simulink model "Kalman_Filter_Simulink_Example"  (R2018a)
settings: Solver=FixedStepAuto  StartTime=0.0  StopTime=30  FixedStep=.01  RelTol=1e-3
values from neighbouring files (symbols this model uses):
  g = 9.81    [Kalman_Filter_Simulink_Example_params.m]
  l = 0.5    [Kalman_Filter_Simulink_Example_params.m]
  P0 = [1e-6 0; 0 1e-6]    [Kalman_Filter_Simulink_Example_params.m]
  Q = 1e-4    (= 0.0001)    [Kalman_Filter_Simulink_Example_params.m]
  R = 1e-3    (= 0.001)    [Kalman_Filter_Simulink_Example_params.m]
  theta0 = pi/4    (= 0.785398163397)    [Kalman_Filter_Simulink_Example_params.m]
  Ts = 0.01    [Kalman_Filter_Simulink_Example_params.m]
undefined symbols (not defined in the file or in its folder): Q0, R0
libraries: simulink x7, dspmtrx3 x5, sharedTrackingLibrary x1, Meldas_Library x1
settings Model: Creator=mulusoy  LastModifiedBy=hussein
settings OptimizationCC: DefaultParameterBehavior=Inlined  PassReuseOutputArgsAs=Individual arguments
settings DebuggingCC: ParameterTunabilityLossMsg=error
settings SFSimCC: MATLABDynamicMemAlloc=off
settings RTWCC: SystemTargetFile=ert.tlc  TemplateMakefile=ert_default_tmf  GenerateReport=on  IncludeHyperlinkInReport=on  LaunchReport=on  GenerateTraceInfo=on  GenerateTraceReport=on  GenerateTraceReportSl=on  GenerateTraceReportSf=on  GenerateTraceReportEml=on  CheckMdlBeforeBuild=Warning
settings CodeAppCC: GenerateComments=off  IgnoreCustomStorageClasses=off  SimulinkBlockComments=off
settings ERTTargetCC: TargetLangStandard=C99 (ISO)  GenerateSampleERTMain=on  InlinedParameterPlacement=NonHierarchical  ERTCustomFileTemplate=example_file_process.tlc
settings SimscapeCC: SimscapeNormalizeSystem=off

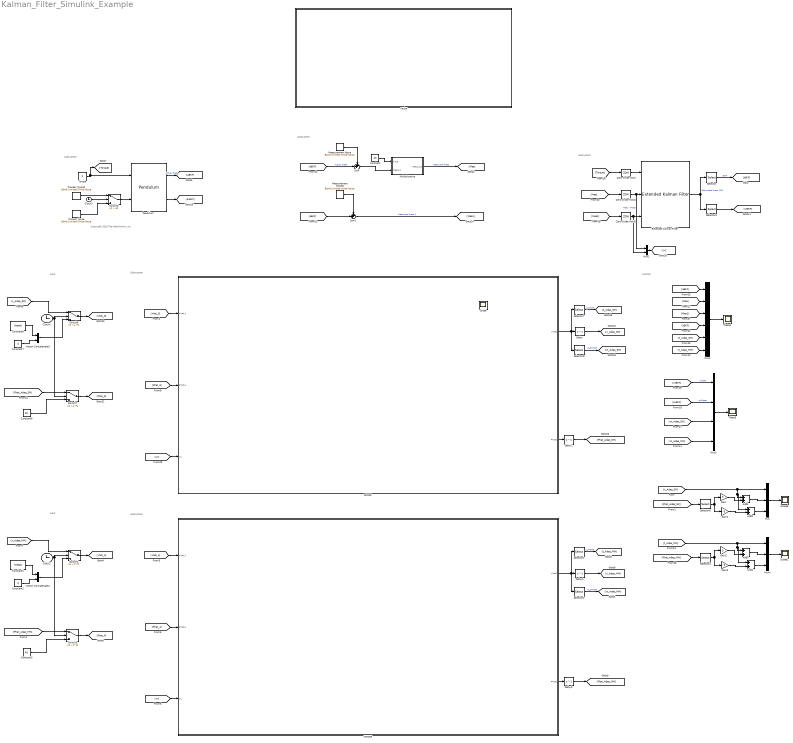
== system Kalman_Filter_Simulink_Example ==
  note: Subsystem
  note: Subsystem
  note: Subsystem
  note: Monitor
  note: Input
  note: Subsystem
  note: Input
  note: Subsystem
  note: Copyright 2018 The MathWorks, Inc.
  Add{1..4} (4 alike) : Sum
  Clock2 : Clock
      settings: Decimation=1000
  Clock3 : Clock
  Clock4 : Clock
      settings: Decimation=1000
  Constant : Constant  Value=20
  Constant1 : Constant  Value=theta0
  Constant2 : Constant  Value=0
  Constant3 : Constant  Value=P0
  Constant6 : Constant  Value=theta0
  Constant7 : Constant  Value=0
  Constant8 : Constant  Value=P0
  Delay{,1..3} (4 alike) : Delay  DelayLength=1
  Extended Kalman Filter : sharedTrackingLibrary/Extended Kalman Filter  StateTransitionFcn=myStateTransitionFcn  HasStateTransitionJacobianFcn=off  HasAdditiveProcessNoise=Additive  ProcessNoise=diag([0,Q0])  HasTimeVaryingProcessNoise=off  HasStateTransitionFcnExtraArgument=1  InitialState=[pi/4 0]  InitialStateCovariance=1e-6  MeasurementFcn1=myMeasurementFcn  HasMeasurementJacobianFcn1=off  HasMeasurementEnablePort1=off  HasAdditiveMeasurementNoise1=Additive  MeasurementNoise1=R0  HasTimeVaryingMeasurementNoise1=off  HasMeasurementFcnExtraArgument1=0  MeasurementFcn2=myMeasurementFcn  HasMeasurementJacobianFcn2=off  HasMeasurementEnablePort2=off  HasAdditiveMeasurementNoise2=Additive  MeasurementNoise2=R0  HasTimeVaryingMeasurementNoise2=off  HasMeasurementFcnExtraArgument2=0  MeasurementFcn3=myMeasurementFcn  HasMeasurementJacobianFcn3=off  HasMeasurementEnablePort3=off  HasAdditiveMeasurementNoise3=Additive  MeasurementNoise3=1  HasTimeVaryingMeasurementNoise3=off  HasMeasurementFcnExtraArgument3=0  MeasurementFcn4=myMeasurementFcn  HasMeasurementJacobianFcn4=off  HasMeasurementEnablePort4=off  HasAdditiveMeasurementNoise4=Additive  MeasurementNoise4=1  HasTimeVaryingMeasurementNoise4=off  HasMeasurementFcnExtraArgument4=0  MeasurementFcn5=myMeasurementFcn  HasMeasurementJacobianFcn5=off  HasMeasurementEnablePort5=off  HasAdditiveMeasurementNoise5=Additive  MeasurementNoise5=1  HasTimeVaryingMeasurementNoise5=off  HasMeasurementFcnExtraArgument5=0  EnableMultirate=off  StateTransitionFcnSampleTime=1  MeasurementFcn1SampleTime=1  MeasurementFcn2SampleTime=1  MeasurementFcn3SampleTime=1  MeasurementFcn4SampleTime=1  MeasurementFcn5SampleTime=1  UseCurrentEstimator=on  OutputStateCovariance=off  DataType=double  SampleTime=Ts  NumberOfMeasurements=2
      settings: SourceProductName=Control System Toolbox  SourceProductBaseCode=CT
  Faults : Subsystem
  Gain : Gain  Gain=3
  Gain1 : Gain  Gain=-3
  Gain2 : Gain  Gain=3
  Gain3 : Gain  Gain=-3
  MMNSF : Subsystem
  Measurement Noise : simulink/Sources/Band-Limited White Noise  Cov=R*Ts  Ts=Ts  seed=[12347]
  Measurement Noise3 : simulink/Sources/Band-Limited White Noise  Cov=R*Ts  Ts=Ts  seed=[12347]
  Multiplicative : Subsystem
  Mux : Mux  Inputs=3
  Mux1 : Mux  Inputs=2
  Mux2 : Mux  Inputs=6
  Mux3 : Mux
  Mux4 : Mux  Inputs=3
  Pendulum : Meldas_Library/Pendulum  theta_0=pi/3  theta_dot_0=0
      link override Revolute Joint: SenseVelocity=on
  Process Noise2 : simulink/Sources/Band-Limited White Noise  Cov=Q*Ts*1000  Ts=Ts  seed=[12347]
  Process Noise : simulink/Sources/Band-Limited White Noise  Cov=0  Ts=Ts  seed=[23341]
  SMNSF : Subsystem
  Scope1 : Scope
  Scope5 : Scope
  Selector : Selector  InputPortWidth=2  IndexOptions=Index vector (dialog)  Indices=1  OutputSizes=1
  Selector1 : Selector  InputPortWidth=2  IndexOptions=Index vector (dialog)  Indices=1  OutputSizes=1
  Selector2 : Selector  InputPortWidth=2  IndexOptions=Index vector (dialog)  Indices=2  OutputSizes=1
  Selector3 : Selector  InputPortWidth=2  IndexOptions=Index vector (dialog)  Indices=2  OutputSizes=1
  Selector4 : Selector  NumberOfDimensions=2  InputPortWidth=3  IndexOptions=Index vector (dialog),Index vector (dialog)  Indices=1,1  OutputSizes=1,1
  Selector6 : Selector  NumberOfDimensions=2  InputPortWidth=3  IndexOptions=Index vector (dialog),Index vector (dialog)  Indices=1,1  OutputSizes=1,1
  Selector7 : Selector  InputPortWidth=2  IndexOptions=Index vector (dialog)  Indices=1  OutputSizes=1
  Selector8 : Selector  InputPortWidth=2  IndexOptions=Index vector (dialog)  Indices=2  OutputSizes=1
  Sum : Sum  Inputs=++|
  Sum1 : Sum  Inputs=++|
  Switch{1,3,6..7} (4 alike) : Switch  Threshold=Ts
  Switch5 : Switch  Criteria=u2 > Threshold  Threshold=40
  Theta4 : Scope
  Theta5 : Scope
  Torque : Constant  Value=0
  Vector Concatenate1 : Concatenate
  Vector Concatenate2 : Concatenate
  Zero-Order Hold : ZeroOrderHold  SampleTime=Ts
  Zero-Order Hold1 : ZeroOrderHold  SampleTime=Ts
  Zero-Order Hold2 : ZeroOrderHold  SampleTime=Ts
  Scope : Scope
  wires:
  [Mea] -> Mux2/2
  [vtEKF] -> Mux3/1  "vtheta"
  Mux3/1 -> Theta5/1
  Mux2/1 -> Theta4/1
  [avEKF] -> Mux3/2  "aVtheta"
  [tEKF] -> Mux2/4
  [aEKF] -> Mux2/1
  [Phat_Adap_SM] -> Selector6/1
  [t_Adap_SM] -> Add2/1, Add1/1, Mux/1
  Selector6/1 -> Gain/1, Gain1/1
  Gain/1 -> Add1/2
  Add1/1 -> Mux/2
  Gain1/1 -> Add2/2
  Add2/1 -> Mux/3
  Mux/1 -> Scope5/1
  Selector7/1 -> [t_Adap_SM]  "t_SMNSF"
  Vector Concatenate2/1 -> Switch6/3
  SMNSF/2(Phat1) -> Delay1/1
  Clock4/1 -> Switch7/2, Switch6/2
  Constant7/1 -> Vector Concatenate2/2
  [x_Adap_SM] -> Switch6/1
  SMNSF/1(xhat1) -> Selector8/1, Selector7/1, Delay/1
  [Phat_3] -> SMNSF/2(Phat_1)
  Constant6/1 -> Vector Concatenate2/1
  [Phat_Adap_SM] -> Switch7/1
  Switch6/1 -> [xhat_3]
  Constant8/1 -> Switch7/3
  Selector8/1 -> [vt_Adap_SM]  "vt_SMNSF"
  Switch7/1 -> [Phat_3]
  [yv] -> SMNSF/3(y1)
  [xhat_3] -> SMNSF/1(xhat_1)
  [t_Adap_SM] -> Mux2/5
  Delay/1 -> [x_Adap_SM]
  Delay1/1 -> [Phat_Adap_SM]
  [Mea1] -> Mux2/3
  [vt_Adap_SM] -> Mux3/3
  Selector1/1 -> [t_Adap_MM]  "t_SMNSF"
  Delay2/1 -> [x_Adap_MM]
  MMNSF/2(Phat1) -> Delay3/1
  Vector Concatenate1/1 -> Switch1/3
  [xhat_4] -> MMNSF/1(xhat_1)
  Selector2/1 -> [vt_Adap_MM]  "vt_SMNSF"
  Switch1/1 -> [xhat_4]
  Constant3/1 -> Switch3/3
  Switch3/1 -> [Phat_4]
  [Phat_4] -> MMNSF/2(Phat_1)
  Constant1/1 -> Vector Concatenate1/1
  [Phat_Adap_MM] -> Switch3/1
  MMNSF/1(xhat1) -> Selector2/1, Selector1/1, Delay2/1
  [x_Adap_MM] -> Switch1/1
  Clock2/1 -> Switch3/2, Switch1/2
  Constant2/1 -> Vector Concatenate1/2
  [yv] -> MMNSF/3(y1)
  Delay3/1 -> [Phat_Adap_MM]
  [t_Adap_MM] -> Mux2/6
  [vt_Adap_MM] -> Mux3/4
  [aEKF] -> Sum/2  "Actual theta"
  [aEKF] -> Sum1/2
  Measurement Noise/1 -> Sum/1
  Measurement Noise3/1 -> Sum1/1
  Sum1/1 -> [Mea1]  "Measured theta 2"
  Multiplicative/1(Meas_out) -> [Mea]  "Measured theta"
  Clock3/1 -> Switch5/2
  Process Noise/1 -> Switch5/3
  Pendulum/2 -> [avEKF]
  Pendulum/1 -> [aEKF]  "Actual theta"
  Torque/1 -> Pendulum/1, [Torque]
  Switch5/1 -> Pendulum/2
  [Mea1] -> Zero-Order Hold2/1
  [Torque] -> Zero-Order Hold/1
  Selector/1 -> [tEKF]  "tEKF"
  Zero-Order Hold/1 -> Extended Kalman Filter/1
  Mux1/1 -> [yv]
  Selector3/1 -> [vtEKF]
  Zero-Order Hold2/1 -> Mux1/2, Extended Kalman Filter/3
  Extended Kalman Filter/1 -> Selector/1, Selector3/1  "Estimated theta  EKF"
  [Mea] -> Zero-Order Hold1/1
  Zero-Order Hold1/1 -> Mux1/1, Extended Kalman Filter/2  "Meas  Theta"
  Process Noise2/1 -> Switch5/1
  Selector4/1 -> Gain2/1, Gain3/1
  Add3/1 -> Mux4/2
  Gain3/1 -> Add4/2
  [Phat_Adap_MM] -> Selector4/1
  [t_Adap_MM] -> Add4/1, Add3/1, Mux4/1
  Gain2/1 -> Add3/2
  Add4/1 -> Mux4/3
  Mux4/1 -> Scope1/1
  Constant/1 -> Multiplicative/1(Time)
  Sum/1 -> Multiplicative/2("Meas_in ")

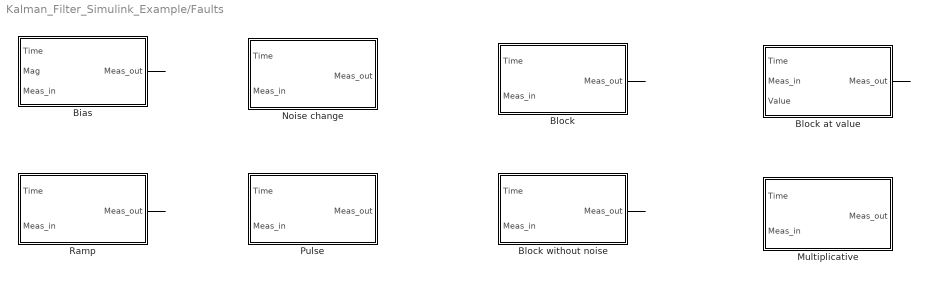
== system Kalman_Filter_Simulink_Example/Faults ==
  Bias : Subsystem
  Block : Subsystem
  Block at value : Subsystem
  Block without noise : Subsystem
  Multiplicative : Subsystem
  Noise change : Subsystem
  Pulse : Subsystem
  Ramp : Subsystem
  wires:
  ? -> Block/2("Meas_in ")
  ? -> Block at value/2("Meas_in ")
  Bias/1(Meas_out) -> ?
  ? -> Ramp/2("Meas_in ")
  ? -> Block without noise/2("Meas_in ")
  Block at value/1(Meas_out) -> ?
  ? -> Bias/1(Time)
  ? -> Block at value/1(Time)
  ? -> Bias/2(Mag)
  Block/1(Meas_out) -> ?
  ? -> Block at value/3(Value)
  Block without noise/1(Meas_out) -> ?
  ? -> Block/1(Time)
  ? -> Block without noise/1(Time)
  Ramp/1(Meas_out) -> ?
  ? -> Ramp/1(Time)
  ? -> Bias/3("Meas_in ")

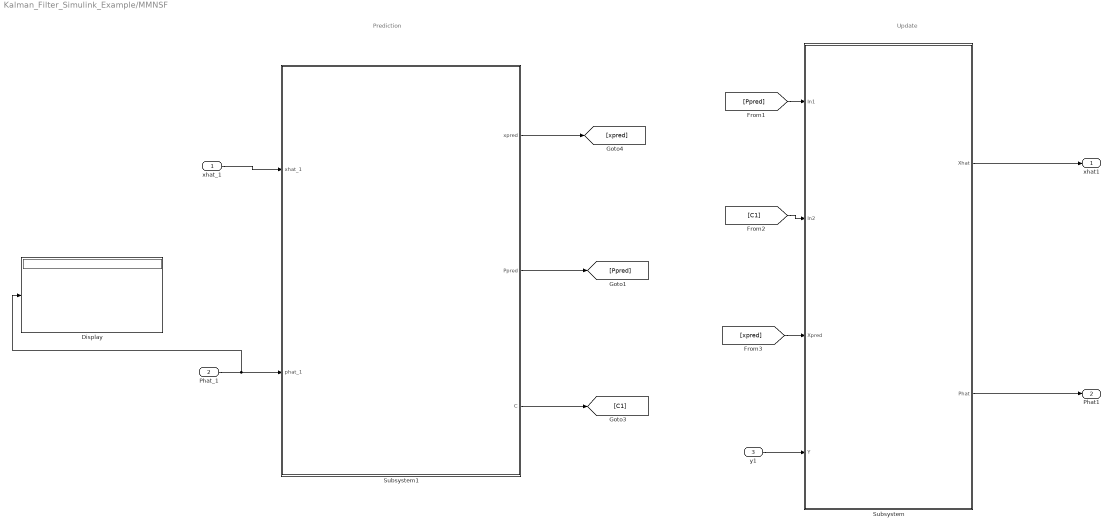
== system Kalman_Filter_Simulink_Example/MMNSF ==
  note: Update
  note: Prediction
  xhat_1 : Inport
  Phat_1 : Inport  Port=2
  y1 : Inport  Port=3
  Display : Display
  Subsystem : Subsystem
  Subsystem1 : Subsystem
  xhat1 : Outport
  Phat1 : Outport  Port=2
  wires:
  [Ppred] -> Subsystem/1(In1)
  Subsystem/1(Xhat) -> xhat1/1
  y1/1 -> Subsystem/4("Y ")
  Subsystem1/1(xpred) -> [xpred]
  Subsystem/2("Phat ") -> Phat1/1
  [C1] -> Subsystem/2(In2)
  Phat_1/1 -> Subsystem1/2(phat_1), Display/1
  [xpred] -> Subsystem/3(Xpred)
  xhat_1/1 -> Subsystem1/1(xhat_1)
  Subsystem1/2(Ppred) -> [Ppred]
  Subsystem1/3("C ") -> [C1]

== system Kalman_Filter_Simulink_Example/Multiplicative ==
  Time : Inport
  "Meas_in " : Inport  Port=2
  Clock : Clock
  Gain : Gain  Gain=2
  Sum : Sum  Inputs=+-
  Switch : Switch  Criteria=u2 > Threshold
  Meas_out : Outport
  wires:
  Switch/1 -> Meas_out/1
  Sum/1 -> Switch/2
  Clock/1 -> Sum/1
  Time/1 -> Sum/2
  "Meas_in "/1 -> Gain/1, Switch/3
  Gain/1 -> Switch/1

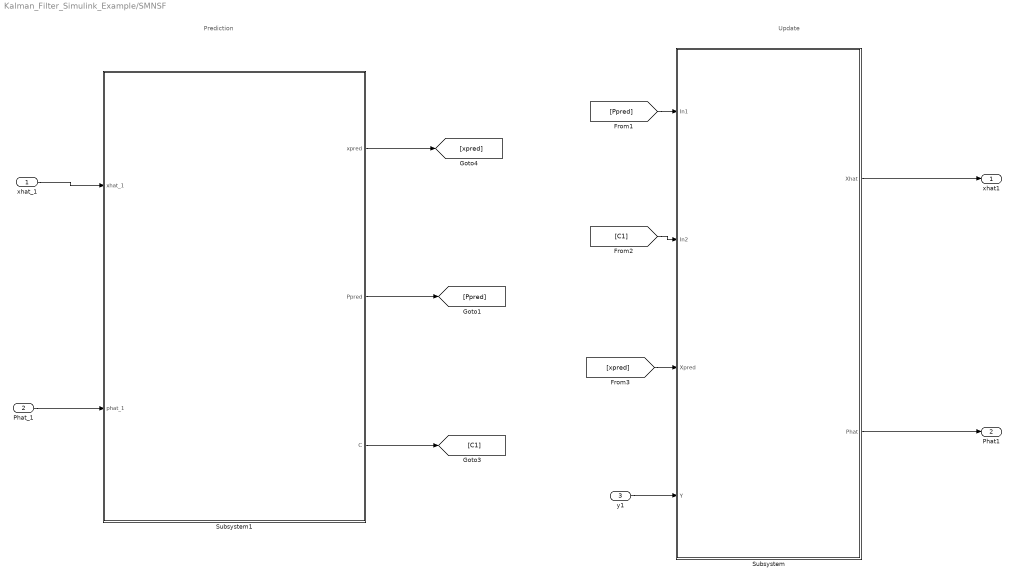
== system Kalman_Filter_Simulink_Example/SMNSF ==
  note: Update
  note: Prediction
  xhat_1 : Inport
  Phat_1 : Inport  Port=2
  y1 : Inport  Port=3
  Subsystem : Subsystem
  Subsystem1 : Subsystem
  xhat1 : Outport
  Phat1 : Outport  Port=2
  wires:
  [Ppred] -> Subsystem/1(In1)
  Subsystem/1(Xhat) -> xhat1/1
  y1/1 -> Subsystem/4("Y ")
  Subsystem1/1(xpred) -> [xpred]
  Subsystem/2("Phat ") -> Phat1/1
  [C1] -> Subsystem/2(In2)
  Phat_1/1 -> Subsystem1/2(phat_1)
  [xpred] -> Subsystem/3(Xpred)
  xhat_1/1 -> Subsystem1/1(xhat_1)
  Subsystem1/2(Ppred) -> [Ppred]
  Subsystem1/3("C ") -> [C1]

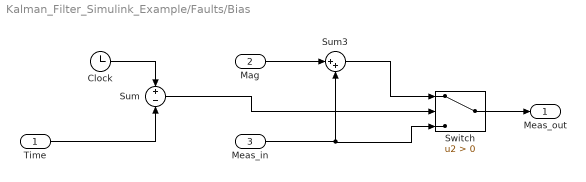
== system Kalman_Filter_Simulink_Example/Faults/Bias ==
  Time : Inport
  Mag : Inport  Port=2
  "Meas_in " : Inport  Port=3
  Clock : Clock
  Sum : Sum  Inputs=+-
  Sum3 : Sum  Inputs=|++
  Switch : Switch  Criteria=u2 > Threshold
  Meas_out : Outport
  wires:
  Sum/1 -> Switch/2
  Clock/1 -> Sum/1
  Switch/1 -> Meas_out/1
  Time/1 -> Sum/2
  Sum3/1 -> Switch/1
  Mag/1 -> Sum3/1
  "Meas_in "/1 -> Sum3/2, Switch/3

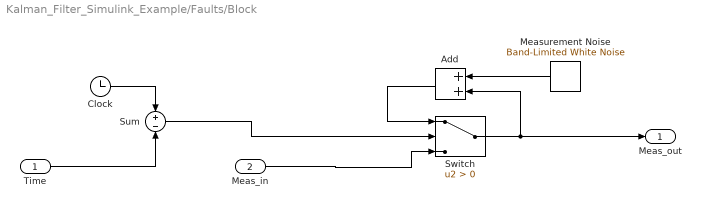
== system Kalman_Filter_Simulink_Example/Faults/Block ==
  Time : Inport
  "Meas_in " : Inport  Port=2
  Add : Sum
  Clock : Clock
  Measurement Noise : simulink/Sources/Band-Limited White Noise  Cov=R*Ts  Ts=Ts  seed=[12347]
  Sum : Sum  Inputs=+-
  Switch : Switch  Criteria=u2 > Threshold
  Meas_out : Outport
  wires:
  "Meas_in "/1 -> Switch/3
  Time/1 -> Sum/2
  Switch/1 -> Add/2, Meas_out/1
  Clock/1 -> Sum/1
  Sum/1 -> Switch/2
  Add/1 -> Switch/1
  Measurement Noise/1 -> Add/1

== system Kalman_Filter_Simulink_Example/Faults/Block at value ==
  Time : Inport
  "Meas_in " : Inport  Port=2
  Value : Inport  Port=3
  Clock : Clock
  Sum : Sum  Inputs=+-
  Switch : Switch  Criteria=u2 > Threshold
  Meas_out : Outport
  wires:
  "Meas_in "/1 -> Switch/3
  Time/1 -> Sum/2
  Clock/1 -> Sum/1
  Sum/1 -> Switch/2
  Switch/1 -> Meas_out/1
  Value/1 -> Switch/1

== system Kalman_Filter_Simulink_Example/Faults/Block without noise ==
  Time : Inport
  "Meas_in " : Inport  Port=2
  Clock : Clock
  Sum : Sum  Inputs=+-
  Switch : Switch  Criteria=u2 > Threshold
  Meas_out : Outport
  wires:
  Switch/1 -> Switch/1, Meas_out/1
  Sum/1 -> Switch/2
  Clock/1 -> Sum/1
  Time/1 -> Sum/2
  "Meas_in "/1 -> Switch/3

== system Kalman_Filter_Simulink_Example/Faults/Multiplicative ==
  Time : Inport
  "Meas_in " : Inport  Port=2
  Clock : Clock
  Gain : Gain  Gain=1.1
  Sum : Sum  Inputs=+-
  Switch : Switch  Criteria=u2 > Threshold
  Meas_out : Outport
  wires:
  Switch/1 -> Meas_out/1
  Sum/1 -> Switch/2
  Clock/1 -> Sum/1
  Time/1 -> Sum/2
  "Meas_in "/1 -> Gain/1, Switch/3
  Gain/1 -> Switch/1

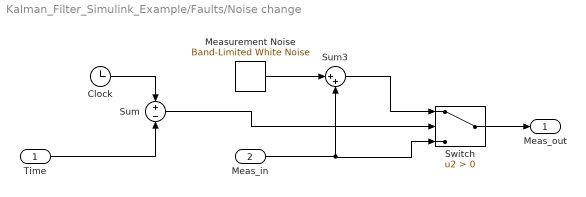
== system Kalman_Filter_Simulink_Example/Faults/Noise change ==
  Time : Inport
  "Meas_in " : Inport  Port=2
  Clock : Clock
  Measurement Noise : simulink/Sources/Band-Limited White Noise  Cov=0.01  Ts=Ts  seed=[12347]
  Sum : Sum  Inputs=+-
  Sum3 : Sum  Inputs=|++
  Switch : Switch  Criteria=u2 > Threshold
  Meas_out : Outport
  wires:
  "Meas_in "/1 -> Switch/3, Sum3/2
  Measurement Noise/1 -> Sum3/1
  Sum3/1 -> Switch/1
  Time/1 -> Sum/2
  Switch/1 -> Meas_out/1
  Clock/1 -> Sum/1
  Sum/1 -> Switch/2

== system Kalman_Filter_Simulink_Example/Faults/Pulse ==
  Time : Inport
  "Meas_in " : Inport  Port=2
  Clock : Clock
  Pulse Generator : DiscretePulseGenerator  Amplitude=0.1  Period=10  PulseWidth=5  SampleTime=0.01
  Sum : Sum  Inputs=+-
  Sum3 : Sum  Inputs=|++
  Switch : Switch  Criteria=u2 > Threshold
  Meas_out : Outport
  wires:
  Sum/1 -> Switch/2
  Clock/1 -> Sum/1
  Switch/1 -> Meas_out/1
  Time/1 -> Sum/2
  Sum3/1 -> Switch/1
  Pulse Generator/1 -> Sum3/1
  "Meas_in "/1 -> Sum3/2, Switch/3

== system Kalman_Filter_Simulink_Example/Faults/Ramp ==
  Time : Inport
  "Meas_in " : Inport  Port=2
  Clock : Clock
  Ramp : simulink/Sources/Ramp  slope=0.1  start=10  InitialOutput=0
  Sum : Sum  Inputs=+-
  Sum3 : Sum  Inputs=|++
  Switch : Switch  Criteria=u2 > Threshold
  Meas_out : Outport
  wires:
  "Meas_in "/1 -> Switch/3, Sum3/2
  Ramp/1 -> Sum3/1
  Sum3/1 -> Switch/1
  Time/1 -> Sum/2
  Switch/1 -> Meas_out/1
  Clock/1 -> Sum/1
  Sum/1 -> Switch/2

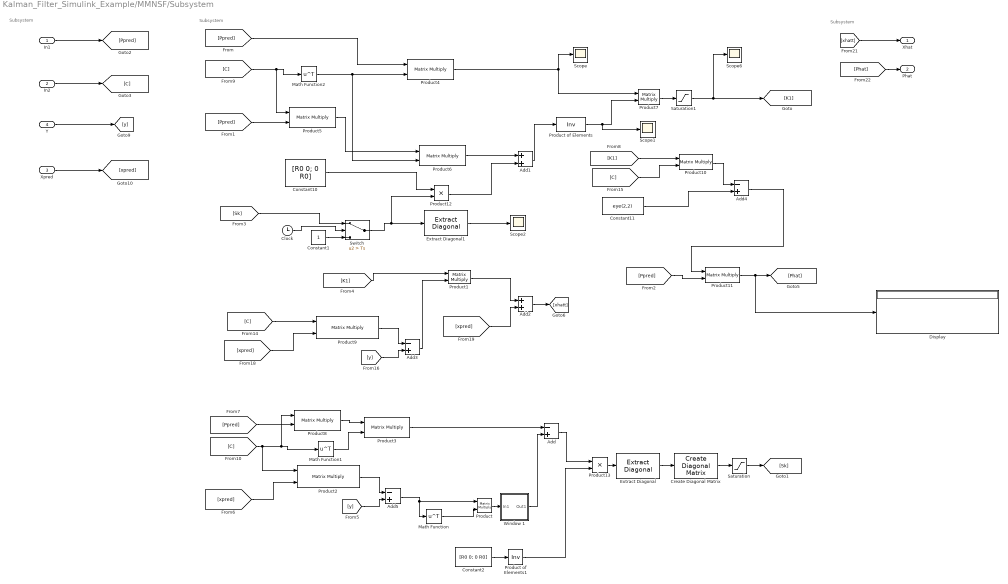
== system Kalman_Filter_Simulink_Example/MMNSF/Subsystem ==
  note: Subsystem
  note: Subsystem
  note: Subsystem
  In1 : Inport
  In2 : Inport  Port=2
  Xpred : Inport  Port=3
  "Y " : Inport  Port=4
  Add{,3..5} (4 alike) : Sum  Inputs=-+
  Add1 : Sum
  Add2 : Sum
  Clock : Clock
  Constant1 : Constant
  Constant10 : Constant  Value=[R0 0; 0 R0]
  Constant11 : Constant  Value=eye(2,2)
  Constant2 : Constant  Value=[R0 0; 0 R0]
  Create Diagonal Matrix : dspmtrx3/Create Diagonal Matrix
      settings: SourceProductName=DSP System Toolbox  SourceProductBaseCode=DS
  Display : Display
  Extract Diagonal : dspmtrx3/Extract Diagonal
      settings: SourceProductName=DSP System Toolbox  SourceProductBaseCode=DS
  Extract Diagonal1 : dspmtrx3/Extract Diagonal
      settings: SourceProductName=DSP System Toolbox  SourceProductBaseCode=DS
  Math Function : Math  Operator=transpose  SaturateOnIntegerOverflow=on
  Math Function1 : Math  Operator=transpose  SaturateOnIntegerOverflow=on
  Math Function2 : Math  Operator=transpose  SaturateOnIntegerOverflow=on
  Product{,1..11} (12 alike) : Product  Multiplication=Matrix(*)
  Product of Elements : Product  Inputs=/  Multiplication=Matrix(*)
  Product of Elements1 : Product  Inputs=/  Multiplication=Matrix(*)
  Product12 : Product
  Product13 : Product
  Saturation : Saturate  UpperLimit=1000  LowerLimit=1
  Saturation1 : Saturate  UpperLimit=1  LowerLimit=0
  Scope{,1..2,6} (4 alike) : Scope
  Switch : Switch  Criteria=u2 > Threshold  Threshold=Ts
  Window 1 : Subsystem
  Xhat : Outport  PortDimensions=[2,1]
  "Phat " : Outport  Port=2
  wires:
  Add2/1 -> [xhatt]
  [K1] -> Product1/1
  [Ppred] -> Product4/1
  Add3/1 -> Product1/2
  Product of Elements/1 -> Scope1/1, Product7/2
  Product5/1 -> Product6/1
  Product9/1 -> Add3/1
  Math Function2/1 -> Product6/2, Product4/2
  Add1/1 -> Product of Elements/1
  Product6/1 -> Add1/1
  Product1/1 -> Add2/1
  [Ppred] -> Product5/2
  [C] -> Product9/1
  [C] -> Product5/1, Math Function2/1
  [y] -> Add3/2
  [xpred] -> Product9/2
  [xpred] -> Add2/2
  In1/1 -> [Ppred]
  In2/1 -> [C]
  Xpred/1 -> [xpred]
  [xhatt] -> Xhat/1
  [Phat] -> "Phat "/1
  Add4/1 -> Product11/1
  [C] -> Product10/2
  Product10/1 -> Add4/1
  [Ppred] -> Product11/2
  [K1] -> Product10/1
  Constant11/1 -> Add4/2
  Product4/1 -> Product7/1, Scope/1
  Constant10/1 -> Product12/1
  Product11/1 -> Display/1, [Phat]
  Product2/1 -> Add5/1
  [xpred] -> Product2/2
  [C] -> Product2/1, Product8/1, Math Function1/1
  [y] -> Add5/2
  Add5/1 -> Math Function/1, Product/1
  Math Function/1 -> Product/2
  [Ppred] -> Product8/2
  Product8/1 -> Product3/1
  Math Function1/1 -> Product3/2
  Product3/1 -> Add/1
  Add/1 -> Product13/1
  Constant2/1 -> Product of Elements1/1
  Product13/1 -> Extract Diagonal/1
  Product12/1 -> Add1/2
  Constant1/1 -> Switch/3
  Clock/1 -> Switch/2
  Switch/1 -> Product12/2, Extract Diagonal1/1
  Product7/1 -> Saturation1/1
  "Y "/1 -> [y]
  Saturation1/1 -> Scope6/1, [K1]
  [Sk] -> Switch/1
  Product/1 -> Window 1/1(In1)
  Window 1/1(Out1) -> Add/2
  Product of Elements1/1 -> Product13/2
  Extract Diagonal/1 -> Create Diagonal Matrix/1
  Create Diagonal Matrix/1 -> Saturation/1
  Saturation/1 -> [Sk]
  Extract Diagonal1/1 -> Scope2/1

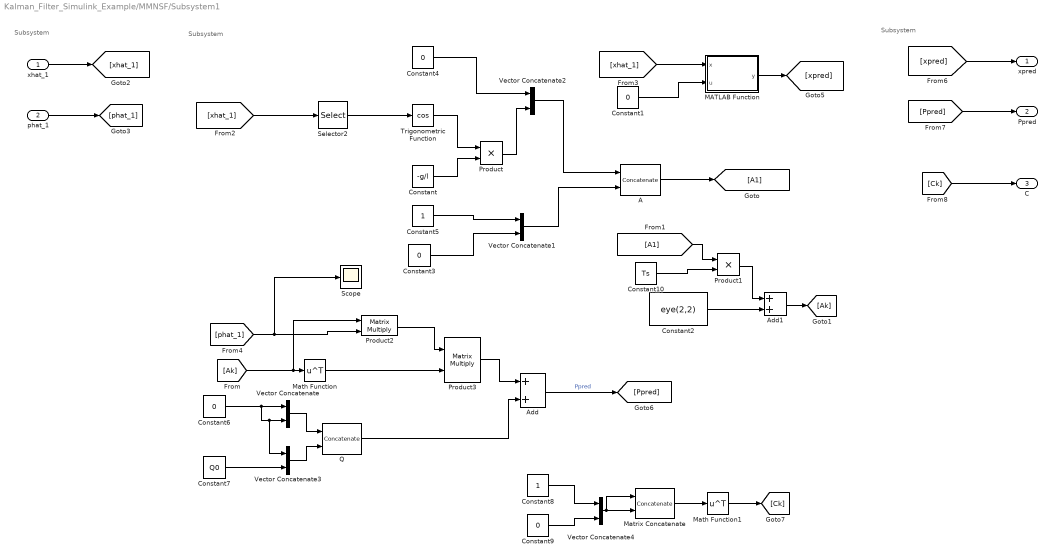
== system Kalman_Filter_Simulink_Example/MMNSF/Subsystem1 ==
  note: Subsystem
  note: Subsystem
  note: Subsystem
  xhat_1 : Inport
  phat_1 : Inport  Port=2
  A : Concatenate  Mode=Multidimensional array  ConcatenateDimension=2
  Add : Sum
  Add1 : Sum
  Constant : Constant  Value=-g/l
  Constant{1,3..4,6,9} (5 alike) : Constant  Value=0
  Constant10 : Constant  Value=Ts
  Constant2 : Constant  Value=eye(2,2)
  Constant5 : Constant
  Constant7 : Constant  Value=Q0
  Constant8 : Constant
  MATLAB Function : MATLAB Function  TreatAsAtomicUnit=on
  Math Function : Math  Operator=transpose  SaturateOnIntegerOverflow=on
  Math Function1 : Math  Operator=transpose  SaturateOnIntegerOverflow=on
  Matrix Concatenate : Concatenate  Mode=Multidimensional array  ConcatenateDimension=2
  Product : Product
  Product1 : Product
  Product2 : Product  Multiplication=Matrix(*)
  Product3 : Product  Multiplication=Matrix(*)
  Q : Concatenate  Mode=Multidimensional array  ConcatenateDimension=2
  Scope : Scope
  Selector2 : Selector  InputPortWidth=2  IndexOptions=Index vector (dialog)  Indices=1  OutputSizes=1
  Trigonometric Function : Trigonometry  Operator=cos
  Vector Concatenate{,1..4} (5 alike) : Concatenate
  xpred : Outport
  Ppred : Outport  Port=2
  "C " : Outport  Port=3
  wires:
  phat_1/1 -> [phat_1]
  xhat_1/1 -> [xhat_1]
  [xpred] -> xpred/1
  [Ppred] -> Ppred/1
  [Ck] -> "C "/1
  Add1/1 -> [Ak]
  Constant2/1 -> Add1/2
  [A1] -> Product1/1
  [xhat_1] -> Selector2/1
  A/1 -> [A1]
  Constant4/1 -> Vector Concatenate2/1
  Constant9/1 -> Vector Concatenate4/2
  Vector Concatenate2/1 -> A/1
  Vector Concatenate4/1 -> Matrix Concatenate/1, Matrix Concatenate/2
  Trigonometric Function/1 -> Product/1
  [phat_1] -> Scope/1, Product2/2
  Product2/1 -> Product3/1
  Constant10/1 -> Product1/2
  [Ak] -> Product2/1, Math Function/1
  Product/1 -> Vector Concatenate2/2
  Selector2/1 -> Trigonometric Function/1
  Vector Concatenate3/1 -> Q/2
  Vector Concatenate1/1 -> A/2
  Product1/1 -> Add1/1
  Math Function/1 -> Product3/2
  Vector Concatenate/1 -> Q/1
  Constant6/1 -> Vector Concatenate3/1, Vector Concatenate/2, Vector Concatenate/1
  Constant1/1 -> MATLAB Function/2(u)
  Constant5/1 -> Vector Concatenate1/1
  Constant3/1 -> Vector Concatenate1/2
  Constant/1 -> Product/2
  Math Function1/1 -> [Ck]
  Product3/1 -> Add/1
  MATLAB Function/1(y) -> [xpred]
  [xhat_1] -> MATLAB Function/1(x)
  Constant8/1 -> Vector Concatenate4/1
  Constant7/1 -> Vector Concatenate3/2
  Add/1 -> [Ppred]  "Ppred"
  Q/1 -> Add/2
  Matrix Concatenate/1 -> Math Function1/1

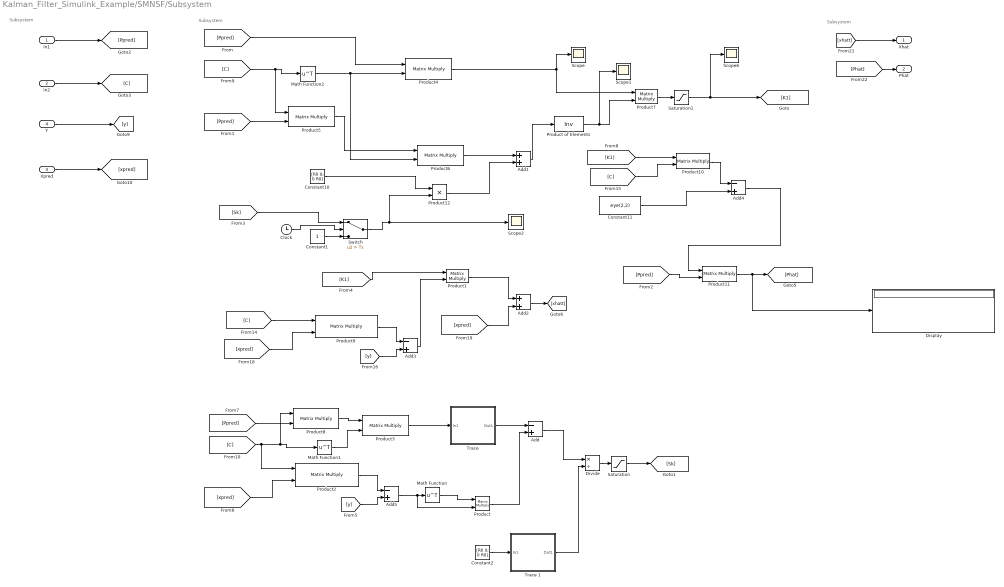
== system Kalman_Filter_Simulink_Example/SMNSF/Subsystem ==
  note: Subsystem
  note: Subsystem
  note: Subsystem
  In1 : Inport
  In2 : Inport  Port=2
  Xpred : Inport  Port=3
  "Y " : Inport  Port=4
  Add{,3..5} (4 alike) : Sum  Inputs=-+
  Add1 : Sum
  Add2 : Sum
  Clock : Clock
  Constant1 : Constant
  Constant10 : Constant  Value=[R0 0; 0 R0]
  Constant11 : Constant  Value=eye(2,2)
  Constant2 : Constant  Value=[R0 0; 0 R0]
  Display : Display
  Divide : Product  Inputs=*/
  Math Function : Math  Operator=transpose  SaturateOnIntegerOverflow=on
  Math Function1 : Math  Operator=transpose  SaturateOnIntegerOverflow=on
  Math Function2 : Math  Operator=transpose  SaturateOnIntegerOverflow=on
  Product{,1..11} (12 alike) : Product  Multiplication=Matrix(*)
  Product of Elements : Product  Inputs=/  Multiplication=Matrix(*)
  Product12 : Product
  Saturation : Saturate  UpperLimit=1000  LowerLimit=1
  Saturation1 : Saturate  UpperLimit=1  LowerLimit=0
  Scope{,1..2,6} (4 alike) : Scope
  Switch : Switch  Criteria=u2 > Threshold  Threshold=Ts
  "Trace " : Subsystem
  Trace 1 : Subsystem
  Xhat : Outport  PortDimensions=[2,1]
  "Phat " : Outport  Port=2
  wires:
  Add2/1 -> [xhatt]
  [K1] -> Product1/1
  [Ppred] -> Product4/1
  Add3/1 -> Product1/2
  Product of Elements/1 -> Scope1/1, Product7/2
  Product5/1 -> Product6/1
  Product9/1 -> Add3/1
  Math Function2/1 -> Product6/2, Product4/2
  Add1/1 -> Product of Elements/1
  Product6/1 -> Add1/1
  Product1/1 -> Add2/1
  [Ppred] -> Product5/2
  [C] -> Product9/1
  [C] -> Product5/1, Math Function2/1
  [y] -> Add3/2
  [xpred] -> Product9/2
  [xpred] -> Add2/2
  In1/1 -> [Ppred]
  In2/1 -> [C]
  Xpred/1 -> [xpred]
  [xhatt] -> Xhat/1
  [Phat] -> "Phat "/1
  Add4/1 -> Product11/1
  [C] -> Product10/2
  Product10/1 -> Add4/1
  [Ppred] -> Product11/2
  [K1] -> Product10/1
  Constant11/1 -> Add4/2
  Product4/1 -> Product7/1, Scope/1
  Constant10/1 -> Product12/1
  Product11/1 -> Display/1, [Phat]
  Product2/1 -> Add5/1
  [xpred] -> Product2/2
  [C] -> Product2/1, Product8/1, Math Function1/1
  [y] -> Add5/2
  Add5/1 -> Product/2, Math Function/1
  Math Function/1 -> Product/1
  Product/1 -> Add/2
  [Ppred] -> Product8/2
  Product8/1 -> Product3/1
  Math Function1/1 -> Product3/2
  Product3/1 -> "Trace "/1(In1)
  "Trace "/1(Out1) -> Add/1
  Add/1 -> Divide/1
  Constant2/1 -> Trace 1/1(In1)
  Trace 1/1(Out1) -> Divide/2
  Divide/1 -> Saturation/1
  Product12/1 -> Add1/2
  Constant1/1 -> Switch/3
  Clock/1 -> Switch/2
  Switch/1 -> Product12/2, Scope2/1
  Saturation/1 -> [Sk]
  Product7/1 -> Saturation1/1
  "Y "/1 -> [y]
  Saturation1/1 -> Scope6/1, [K1]
  [Sk] -> Switch/1

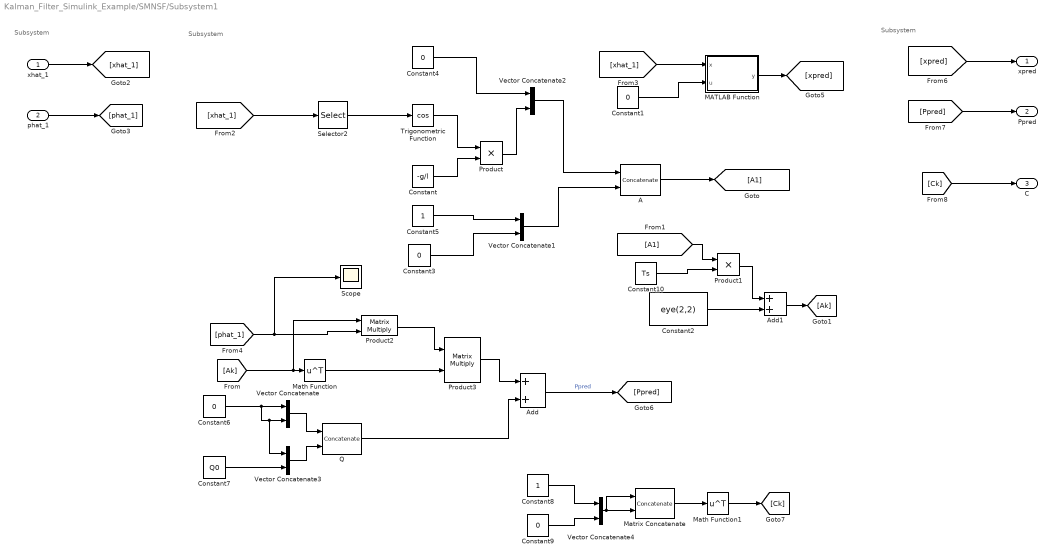
== system Kalman_Filter_Simulink_Example/SMNSF/Subsystem1 ==
  note: Subsystem
  note: Subsystem
  note: Subsystem
  xhat_1 : Inport
  phat_1 : Inport  Port=2
  A : Concatenate  Mode=Multidimensional array  ConcatenateDimension=2
  Add : Sum
  Add1 : Sum
  Constant : Constant  Value=-g/l
  Constant{1,3..4,6,9} (5 alike) : Constant  Value=0
  Constant10 : Constant  Value=Ts
  Constant2 : Constant  Value=eye(2,2)
  Constant5 : Constant
  Constant7 : Constant  Value=Q0
  Constant8 : Constant
  MATLAB Function : MATLAB Function  TreatAsAtomicUnit=on
  Math Function : Math  Operator=transpose  SaturateOnIntegerOverflow=on
  Math Function1 : Math  Operator=transpose  SaturateOnIntegerOverflow=on
  Matrix Concatenate : Concatenate  Mode=Multidimensional array  ConcatenateDimension=2
  Product : Product
  Product1 : Product
  Product2 : Product  Multiplication=Matrix(*)
  Product3 : Product  Multiplication=Matrix(*)
  Q : Concatenate  Mode=Multidimensional array  ConcatenateDimension=2
  Scope : Scope
  Selector2 : Selector  InputPortWidth=2  IndexOptions=Index vector (dialog)  Indices=1  OutputSizes=1
  Trigonometric Function : Trigonometry  Operator=cos
  Vector Concatenate{,1..4} (5 alike) : Concatenate
  xpred : Outport
  Ppred : Outport  Port=2
  "C " : Outport  Port=3
  wires:
  phat_1/1 -> [phat_1]
  xhat_1/1 -> [xhat_1]
  [xpred] -> xpred/1
  [Ppred] -> Ppred/1
  [Ck] -> "C "/1
  Add1/1 -> [Ak]
  Constant2/1 -> Add1/2
  [A1] -> Product1/1
  [xhat_1] -> Selector2/1
  A/1 -> [A1]
  Constant4/1 -> Vector Concatenate2/1
  Constant9/1 -> Vector Concatenate4/2
  Vector Concatenate2/1 -> A/1
  Vector Concatenate4/1 -> Matrix Concatenate/1, Matrix Concatenate/2
  Trigonometric Function/1 -> Product/1
  [phat_1] -> Scope/1, Product2/2
  Product2/1 -> Product3/1
  Constant10/1 -> Product1/2
  [Ak] -> Product2/1, Math Function/1
  Product/1 -> Vector Concatenate2/2
  Selector2/1 -> Trigonometric Function/1
  Vector Concatenate3/1 -> Q/2
  Vector Concatenate1/1 -> A/2
  Product1/1 -> Add1/1
  Math Function/1 -> Product3/2
  Vector Concatenate/1 -> Q/1
  Constant6/1 -> Vector Concatenate3/1, Vector Concatenate/2, Vector Concatenate/1
  Constant1/1 -> MATLAB Function/2(u)
  Constant5/1 -> Vector Concatenate1/1
  Constant3/1 -> Vector Concatenate1/2
  Constant/1 -> Product/2
  Math Function1/1 -> [Ck]
  Product3/1 -> Add/1
  MATLAB Function/1(y) -> [xpred]
  [xhat_1] -> MATLAB Function/1(x)
  Constant8/1 -> Vector Concatenate4/1
  Constant7/1 -> Vector Concatenate3/2
  Add/1 -> [Ppred]  "Ppred"
  Q/1 -> Add/2
  Matrix Concatenate/1 -> Math Function1/1

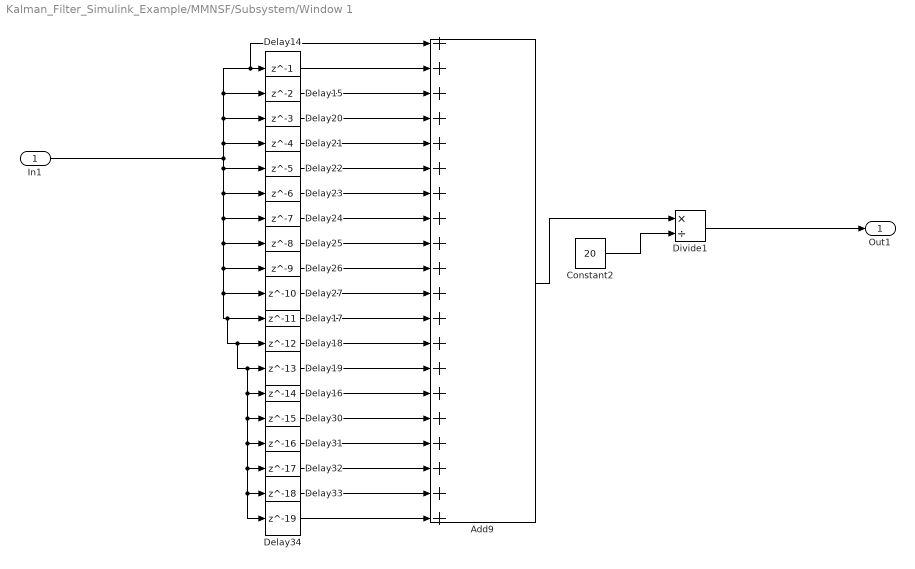
== system Kalman_Filter_Simulink_Example/MMNSF/Subsystem/Window 1 ==
  In1 : Inport
  Add9 : Sum  Inputs=20
  Constant2 : Constant  Value=20
  Delay14 : Delay  DelayLength=1  SampleTime=Ts
  Delay15 : Delay  SampleTime=Ts
  Delay16 : Delay  DelayLength=14  SampleTime=Ts
  Delay17 : Delay  DelayLength=11  SampleTime=Ts
  Delay18 : Delay  DelayLength=12  SampleTime=Ts
  Delay19 : Delay  DelayLength=13  SampleTime=Ts
  Delay20 : Delay  DelayLength=3  SampleTime=Ts
  Delay21 : Delay  DelayLength=4  SampleTime=Ts
  Delay22 : Delay  DelayLength=5  SampleTime=Ts
  Delay23 : Delay  DelayLength=6  SampleTime=Ts
  Delay24 : Delay  DelayLength=7  SampleTime=Ts
  Delay25 : Delay  DelayLength=8  SampleTime=Ts
  Delay26 : Delay  DelayLength=9  SampleTime=Ts
  Delay27 : Delay  DelayLength=10  SampleTime=Ts
  Delay30 : Delay  DelayLength=15  SampleTime=Ts
  Delay31 : Delay  DelayLength=16  SampleTime=Ts
  Delay32 : Delay  DelayLength=17  SampleTime=Ts
  Delay33 : Delay  DelayLength=18  SampleTime=Ts
  Delay34 : Delay  DelayLength=19  SampleTime=Ts
  Divide1 : Product  Inputs=*/
  Out1 : Outport
  wires:
  Delay31/1 -> Add9/17
  Delay30/1 -> Add9/16
  Delay14/1 -> Add9/2
  Add9/1 -> Divide1/1
  Delay17/1 -> Add9/12
  Delay19/1 -> Add9/14
  Delay23/1 -> Add9/7
  Delay25/1 -> Add9/9
  Delay26/1 -> Add9/10
  Delay18/1 -> Add9/13
  Delay24/1 -> Add9/8
  Delay20/1 -> Add9/4
  Delay21/1 -> Add9/5
  Delay15/1 -> Add9/3
  Delay32/1 -> Add9/18
  Delay34/1 -> Add9/20
  Delay33/1 -> Add9/19
  Delay22/1 -> Add9/6
  Constant2/1 -> Divide1/2
  Delay27/1 -> Add9/11
  In1/1 -> Delay14/1, Add9/1, Delay15/1, Delay20/1, Delay21/1, Delay34/1, Delay33/1, Delay32/1, Delay31/1, Delay30/1, Delay16/1, Delay19/1, Delay18/1, Delay17/1, Delay27/1, Delay26/1, Delay25/1, Delay24/1, Delay23/1, Delay22/1
  Delay16/1 -> Add9/15
  Divide1/1 -> Out1/1

== system Kalman_Filter_Simulink_Example/SMNSF/Subsystem/Trace  ==
  In1 : Inport
  Extract Diagonal : dspmtrx3/Extract Diagonal
      settings: SourceProductName=DSP System Toolbox  SourceProductBaseCode=DS
  Sum of Elements : Sum  Inputs=+
  Out1 : Outport
  wires:
  Extract Diagonal/1 -> Sum of Elements/1
  Sum of Elements/1 -> Out1/1
  In1/1 -> Extract Diagonal/1

== system Kalman_Filter_Simulink_Example/SMNSF/Subsystem/Trace 1 ==
  In1 : Inport
  Extract Diagonal : dspmtrx3/Extract Diagonal
      settings: SourceProductName=DSP System Toolbox  SourceProductBaseCode=DS
  Sum of Elements : Sum  Inputs=+
  Out1 : Outport
  wires:
  Extract Diagonal/1 -> Sum of Elements/1
  Sum of Elements/1 -> Out1/1
  In1/1 -> Extract Diagonal/1

== matlab function Kalman_Filter_Simulink_Example/MMNSF/Subsystem1/MATLAB Function ==
  data: x input; u input; y output
function y =Trans(x,u)

dt = 0.01;

y= x + [x(2); -9.81/0.5*sin(x(1))+u]*dt;
end

== matlab function Kalman_Filter_Simulink_Example/SMNSF/Subsystem1/MATLAB Function ==
  data: x input; u input; y output
function y =Trans(x,u)

dt = 0.01;

y= x + [x(2); -9.81/0.5*sin(x(1))+u]*dt;
end
